simulink model "gm_sampleModel1988_1_sub_sub"  (R2023a)
settings: Solver=VariableStepAuto  StartTime=0.0  StopTime=10.0  RelTol=1e-3
libraries: simulink x4, hdlsllib x3
settings Model: Creator=user1  LastModifiedBy=user1
settings OptimizationCC: BlockReduction=off  ConditionallyExecuteInputs=off
settings DebuggingCC: InheritedTsInSrcMsg=none

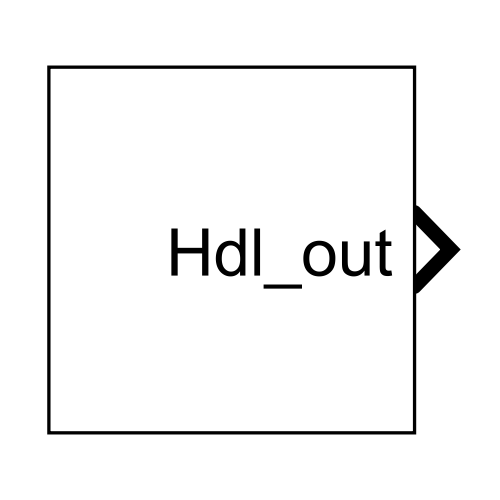
[thumbnail: Simulink's stored preview of the top-level diagram]
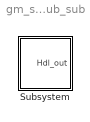
== system gm_sampleModel1988_1_sub_sub ==
  Subsystem : Subsystem

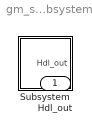
== system gm_sampleModel1988_1_sub_sub/Subsystem ==
  Subsystem : Subsystem
  Hdl_out : Outport  OutDataTypeStr=uint8

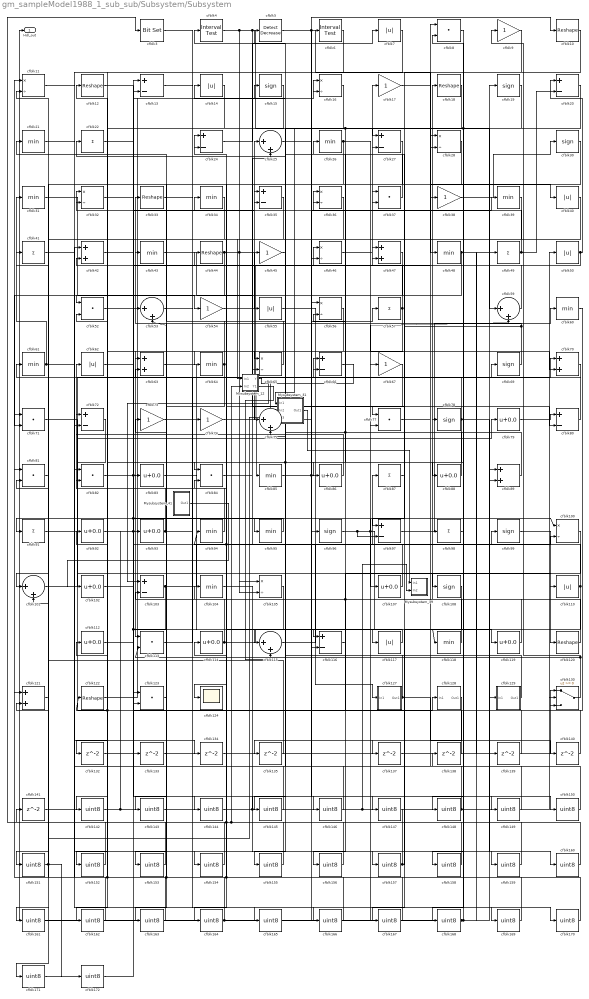
== system gm_sampleModel1988_1_sub_sub/Subsystem/Subsystem ==
  Mysubsystem_12 : Subsystem  TreatAsAtomicUnit=on  RTWFcnName=Mysubsystem_12
      settings: RTWFcnNameOpts=User specified  RTWFileNameOpts=Use function name
  Mysubsystem_31 : Subsystem  TreatAsAtomicUnit=on  RTWFcnName=Mysubsystem_31
      settings: RTWFcnNameOpts=User specified  RTWFileNameOpts=Use function name
  Mysubsystem_39 : Subsystem  TreatAsAtomicUnit=on  RTWFcnName=Mysubsystem_39
      settings: RTWFcnNameOpts=User specified  RTWFileNameOpts=Use function name
  Mysubsystem_41 : Subsystem  TreatAsAtomicUnit=on  RTWFcnName=Mysubsystem_41
      settings: RTWFcnNameOpts=User specified  RTWFileNameOpts=Use function name
  cfblk{10,12,18,33,44,120,122} (7 alike) : Reshape
  cfblk{11,16,28,32,36,46,56,65,100,105} (10 alike) : Product  Inputs=*/  OutDataTypeStr=uint8  RndMeth=Zero  SaturateOnIntegerOverflow=on
  cfblk{25,53,59,75,101,115} (6 alike) : Sum  Inputs=|++  OutDataTypeStr=uint8
  cfblk{79,83,86,88,92..93,102,107,112,114,119} (11 alike) : Bias  Bias=0.0  SaturateOnIntegerOverflow=off
  cfblk{13,20,24,27,35,66,72,80,97,103,116} (11 alike) : Sum  Inputs=+-  OutDataTypeStr=uint8
  cfblk{21,26,31,34,39,43,48,60..61,64,85,94..95,104,118} (15 alike) : MinMax  OutDataTypeStr=uint8
  cfblk{15,19,30,69,78,96,99,108} (8 alike) : Signum
  cfblk{7,14,40,50,55,62,110,117} (8 alike) : Abs  OutDataTypeStr=uint8  SaturateOnIntegerOverflow=off
  cfblk{8,37,52,71,77,81..82,84,113,123} (10 alike) : DotProduct  OutDataTypeStr=uint8
  cfblk{42,47,63,70,89,121} (6 alike) : Sum  OutDataTypeStr=uint8
  cfblk124 : Scope
  cfblk127 : Subsystem
      settings: LibrarySourceBlock=|
      | hdlsllib/Ports &
      | Subsystems/Subsystem
  cfblk128 : Subsystem
      settings: LibrarySourceBlock=|
      | hdlsllib/Ports &
      | Subsystems/Subsystem
  cfblk129 : Subsystem
      settings: LibrarySourceBlock=|
      | hdlsllib/Ports &
      | Subsystems/Subsystem
  cfblk130 : Switch  OutDataTypeStr=uint8  SaturateOnIntegerOverflow=off  InputSameDT=off
  cfblk{132..135,137..141} (9 alike) : Delay  SampleTime=1
  cfblk{142..172} (31 alike) : DataTypeConversion  OutDataTypeStr=uint8  SaturateOnIntegerOverflow=off  RndMeth=Floor
  cfblk{9,17,38,45,54,67,73..74} (8 alike) : Gain  OutDataTypeStr=uint8
  cfblk{22,41,49,57,87,91,98} (7 alike) : Sum  Inputs=+  OutDataTypeStr=uint8
  cfblk3 : simulink/Logic and Bit Operations/Bit Set  iBit=0
      settings: LibrarySourceBlock=|
      | hdlsllib/Logic and Bit
      | Operations/Bit Set
  cfblk4 : hdlsllib/Logic and Bit Operations/Interval Test  IntervalClosedRight=on  uplimit=0.5  IntervalClosedLeft=on  lowlimit=-0.5  OutDataTypeStr=uint8
  cfblk5 : simulink/Logic and Bit Operations/Detect Decrease  vinit=0.0  OutDataTypeStr=uint8
      settings: LibrarySourceBlock=|
      | hdlsllib/Logic and Bit
      | Operations/Detect
      | Decrease
  cfblk6 : hdlsllib/Logic and Bit Operations/Interval Test  IntervalClosedRight=on  uplimit=0.5  IntervalClosedLeft=on  lowlimit=-0.5  OutDataTypeStr=uint8
  Hdl_out : Outport  OutDataTypeStr=uint8
  wires:
  cfblk122/1 -> cfblk16/1
  cfblk119/1 -> cfblk18/1
  cfblk96/1 -> cfblk97/2, cfblk59/2, cfblk119/1
  cfblk56/1 -> cfblk113/1
  cfblk74/1 -> cfblk25/1
  cfblk72/1 -> cfblk128/1(In1)
  cfblk129/1(Out1) -> cfblk14/1
  cfblk5/1 -> cfblk147/1, cfblk10/1, cfblk48/1
  cfblk69/1 -> cfblk37/1, cfblk33/1
  cfblk65/1 -> cfblk21/1
  cfblk114/1 -> cfblk53/1, cfblk117/1
  cfblk46/1 -> cfblk17/1
  cfblk78/1 -> cfblk160/1, cfblk5/1, cfblk152/1, cfblk145/1
  cfblk44/1 -> cfblk71/2, cfblk105/2, cfblk85/1
  cfblk112/1 -> cfblk35/1
  cfblk80/1 -> cfblk61/1
  cfblk107/1 -> cfblk87/1
  cfblk115/1 -> cfblk99/1
  cfblk31/1 -> cfblk54/1
  cfblk82/1 -> cfblk44/1, cfblk46/1
  cfblk99/1 -> cfblk120/1
  cfblk22/1 -> cfblk108/1
  cfblk73/1 -> cfblk166/1
  cfblk105/1 -> cfblk124/1
  cfblk24/1 -> cfblk7/1
  cfblk102/1 -> cfblk70/1
  cfblk95/1 -> cfblk91/1
  cfblk89/1 -> cfblk26/1, cfblk22/1
  cfblk52/1 -> cfblk34/1
  cfblk55/1 -> cfblk127/1(In1)
  cfblk64/1 -> cfblk163/1, cfblk43/1
  cfblk38/1 -> cfblk30/1
  cfblk61/1 -> cfblk134/1, cfblk31/1
  cfblk93/1 -> cfblk66/2, cfblk62/1
  cfblk117/1 -> cfblk115/1
  cfblk63/1 -> cfblk129/1(In1)
  cfblk17/1 -> cfblk40/1
  cfblk15/1 -> cfblk52/1
  cfblk130/1 -> cfblk9/1, cfblk113/2
  cfblk98/1 -> cfblk168/1
  cfblk12/1 -> cfblk144/1
  cfblk34/1 -> cfblk101/1
  cfblk47/1 -> cfblk64/1
  cfblk25/1 -> cfblk96/1
  cfblk118/1 -> cfblk45/1
  cfblk88/1 -> cfblk32/1
  cfblk41/1 -> cfblk157/1
  cfblk101/1 -> cfblk28/1
  cfblk40/1 -> cfblk97/1
  cfblk39/1 -> cfblk75/1
  cfblk48/1 -> cfblk153/1, cfblk139/1
  cfblk71/1 -> cfblk110/1
  cfblk27/1 -> cfblk63/1
  cfblk86/1 -> cfblk72/1
  cfblk97/1 -> cfblk60/1
  cfblk104/1 -> cfblk159/1
  cfblk121/1 -> cfblk151/1
  cfblk37/1 -> cfblk4/1
  cfblk50/1 -> cfblk47/2, cfblk20/1
  cfblk8/1 -> cfblk148/1
  cfblk60/1 -> cfblk130/1
  cfblk30/1 -> cfblk75/2
  cfblk36/1 -> cfblk83/1
  cfblk33/1 -> cfblk74/1
  cfblk91/1 -> cfblk78/1
  cfblk4/1 -> cfblk105/1, cfblk80/2, cfblk59/1
  cfblk54/1 -> cfblk38/1
  cfblk62/1 -> cfblk149/1, cfblk118/1
  cfblk75/1 -> cfblk57/1
  cfblk84/1 -> cfblk47/1
  cfblk6/1 -> cfblk142/1
  cfblk120/1 -> cfblk84/2, cfblk36/1
  cfblk32/1 -> cfblk116/1
  cfblk19/1 -> cfblk158/1, cfblk86/1, Mysubsystem_31/1(In1)
  cfblk92/1 -> cfblk100/2, cfblk16/2, cfblk100/1
  cfblk113/1 -> cfblk79/1
  cfblk67/1 -> cfblk164/1
  cfblk127/1(Out1) -> cfblk140/1, cfblk56/2
  cfblk103/1 -> cfblk123/2, cfblk25/2
  cfblk94/1 -> cfblk32/2
  cfblk85/1 -> cfblk39/1, cfblk107/1
  cfblk83/1 -> cfblk95/1
  cfblk9/1 -> cfblk27/1
  cfblk7/1 -> cfblk72/2
  cfblk16/1 -> cfblk116/2
  cfblk59/1 -> cfblk35/2
  cfblk110/1 -> cfblk137/1, cfblk24/1
  cfblk26/1 -> cfblk70/2, cfblk84/1
  cfblk87/1 -> cfblk27/2
  cfblk57/1 -> cfblk132/1, cfblk42/2
  cfblk13/1 -> cfblk170/1
  cfblk20/1 -> cfblk88/1
  cfblk49/1 -> cfblk20/2, cfblk15/1
  cfblk77/1 -> cfblk69/1
  cfblk10/1 -> cfblk77/1
  cfblk45/1 -> cfblk65/1
  cfblk70/1 -> cfblk63/2
  cfblk116/1 -> cfblk66/1
  cfblk79/1 -> cfblk80/1
  cfblk43/1 -> cfblk65/2
  cfblk132/1 -> cfblk130/2
  cfblk42/1 -> cfblk133/1
  cfblk133/1 -> cfblk46/2
  cfblk134/1 -> cfblk130/3
  cfblk128/1(Out1) -> cfblk135/1
  cfblk135/1 -> cfblk101/2
  cfblk137/1 -> cfblk28/2
  cfblk138/1 -> cfblk123/1
  cfblk139/1 -> cfblk36/2
  cfblk140/1 -> cfblk103/2
  cfblk141/1 -> cfblk89/1
  cfblk142/1 -> cfblk93/1, cfblk89/2
  cfblk123/1 -> cfblk143/1
  cfblk143/1 -> cfblk6/1
  cfblk144/1 -> cfblk150/1, Mysubsystem_39/2(In2), cfblk77/2
  cfblk145/1 -> cfblk12/1
  cfblk3/1 -> cfblk146/1
  cfblk146/1 -> cfblk55/1
  cfblk147/1 -> cfblk3/1
  cfblk148/1 -> cfblk50/1, cfblk42/1
  cfblk149/1 -> cfblk8/1
  cfblk150/1 -> cfblk8/2
  cfblk151/1 -> cfblk172/1, Mysubsystem_31/3(In3)
  cfblk152/1 -> cfblk121/1
  cfblk153/1 -> cfblk121/2
  cfblk11/1 -> cfblk154/1
  cfblk154/1 -> cfblk52/2
  cfblk18/1 -> cfblk155/1
  cfblk155/1 -> cfblk11/1
  cfblk100/1 -> cfblk156/1
  cfblk156/1 -> cfblk11/2
  cfblk157/1 -> cfblk37/2, cfblk71/1, Mysubsystem_12/2(In2)
  cfblk158/1 -> cfblk41/1
  cfblk159/1 -> cfblk92/1, cfblk94/1, cfblk24/2
  cfblk160/1 -> cfblk104/1
  cfblk81/1 -> cfblk161/1
  cfblk161/1 -> cfblk19/1
  cfblk14/1 -> cfblk162/1
  cfblk162/1 -> cfblk81/1
  cfblk163/1 -> cfblk81/2
  cfblk164/1 -> cfblk56/1, cfblk82/2
  cfblk53/1 -> cfblk165/1
  cfblk165/1 -> cfblk67/1
  cfblk166/1 -> cfblk114/1, cfblk53/2, cfblk141/1
  cfblk108/1 -> cfblk167/1
  cfblk167/1 -> cfblk73/1
  cfblk168/1 -> Hdl_out/1, cfblk49/1, cfblk138/1
  cfblk21/1 -> cfblk169/1
  cfblk169/1 -> cfblk98/1
  cfblk170/1 -> cfblk82/1, cfblk122/1, cfblk112/1
  cfblk28/1 -> cfblk171/1
  cfblk171/1 -> cfblk13/1
  cfblk172/1 -> cfblk13/2
  cfblk35/1 -> Mysubsystem_12/1(In1)
  Mysubsystem_12/1(Y) -> cfblk103/1
  Mysubsystem_12/2(Y1) -> cfblk115/2
  cfblk66/1 -> Mysubsystem_31/2(In2)
  Mysubsystem_31/1(Out1) -> Mysubsystem_39/1(In1)
  Mysubsystem_41/1(Out1) -> cfblk102/1

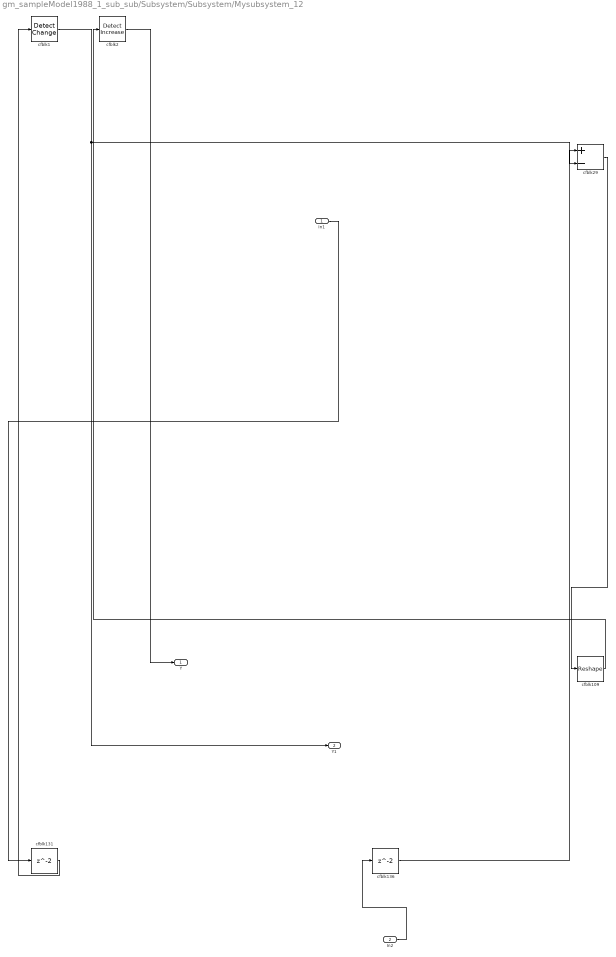
== system gm_sampleModel1988_1_sub_sub/Subsystem/Subsystem/Mysubsystem_12 ==
  In1 : Inport
  In2 : Inport  Port=2
  cfblk1 : simulink/Logic and Bit Operations/Detect Change  vinit=0  OutDataTypeStr=boolean
      settings: LibrarySourceBlock=|
      | hdlsllib/Logic and Bit
      | Operations/Detect
      | Change
  cfblk109 : Reshape
  cfblk131 : Delay  SampleTime=1
  cfblk136 : Delay  SampleTime=1
  cfblk2 : simulink/Logic and Bit Operations/Detect Increase  vinit=0.0  OutDataTypeStr=boolean
      settings: LibrarySourceBlock=|
      | hdlsllib/Logic and Bit
      | Operations/Detect
      | Increase
  cfblk29 : Sum  Inputs=+-
  Y : Outport
  Y1 : Outport  Port=2
  wires:
  In2/1 -> cfblk136/1
  In1/1 -> cfblk131/1
  cfblk136/1 -> cfblk29/1
  cfblk131/1 -> cfblk1/1
  cfblk29/1 -> cfblk109/1
  cfblk1/1 -> cfblk29/2, Y1/1
  cfblk109/1 -> cfblk2/1
  cfblk2/1 -> Y/1

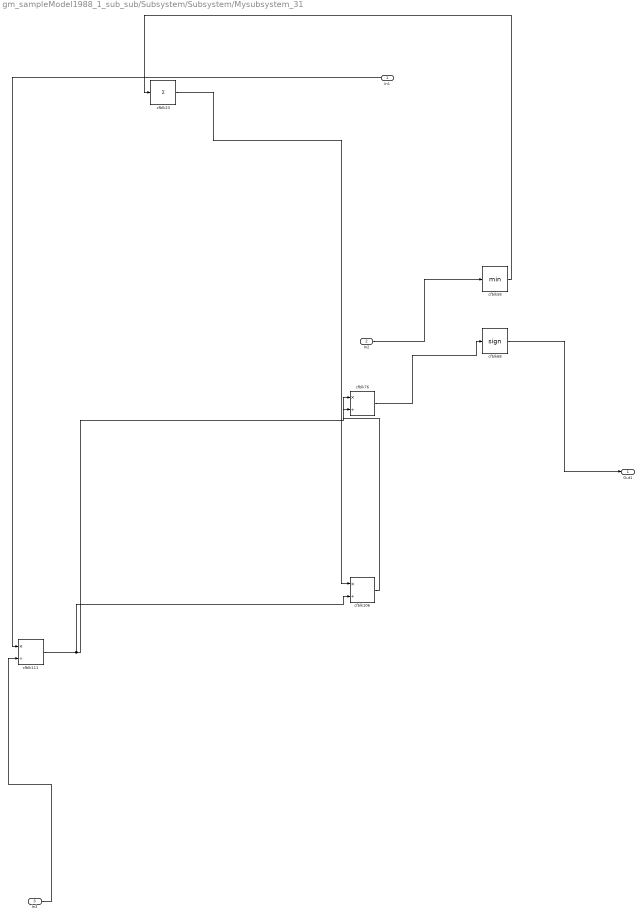
== system gm_sampleModel1988_1_sub_sub/Subsystem/Subsystem/Mysubsystem_31 ==
  In1 : Inport
  In2 : Inport  Port=2
  In3 : Inport  Port=3
  cfblk106 : Product  Inputs=*/  RndMeth=Zero  SaturateOnIntegerOverflow=on
  cfblk111 : Product  Inputs=*/  RndMeth=Zero  SaturateOnIntegerOverflow=on
  cfblk23 : Sum  Inputs=+
  cfblk58 : MinMax
  cfblk68 : Signum
  cfblk76 : Product  Inputs=*/  RndMeth=Zero  SaturateOnIntegerOverflow=on
  Out1 : Outport
  wires:
  In1/1 -> cfblk111/1
  In2/1 -> cfblk58/1
  cfblk68/1 -> Out1/1
  cfblk106/1 -> cfblk76/2
  In3/1 -> cfblk111/2
  cfblk76/1 -> cfblk68/1
  cfblk23/1 -> cfblk106/1
  cfblk58/1 -> cfblk23/1
  cfblk111/1 -> cfblk106/2, cfblk76/1

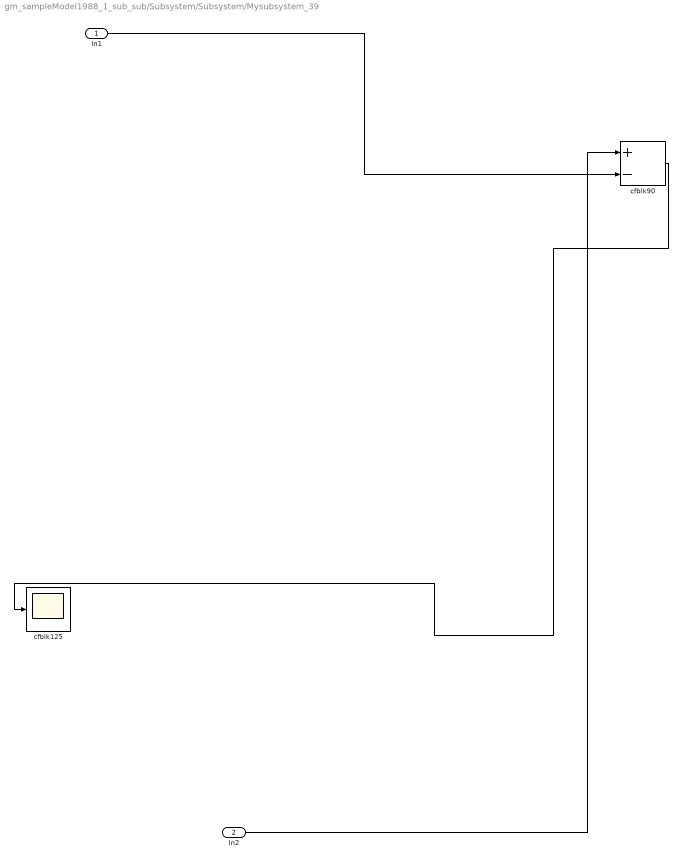
== system gm_sampleModel1988_1_sub_sub/Subsystem/Subsystem/Mysubsystem_39 ==
  In1 : Inport
  In2 : Inport  Port=2
  cfblk125 : Scope
  cfblk90 : Sum  Inputs=+-
  wires:
  In1/1 -> cfblk90/2
  cfblk90/1 -> cfblk125/1
  In2/1 -> cfblk90/1

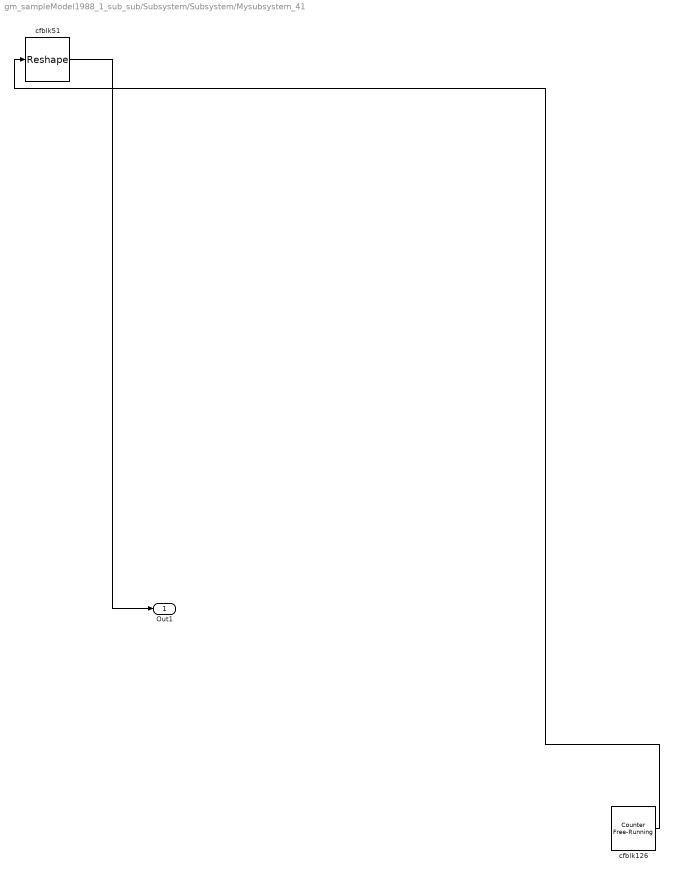
== system gm_sampleModel1988_1_sub_sub/Subsystem/Subsystem/Mysubsystem_41 ==
  cfblk126 : hdlsllib/Sources/Counter Free-Running  NumBits=16  tsamp=-1
  cfblk51 : Reshape
  Out1 : Outport
  wires:
  cfblk51/1 -> Out1/1
  cfblk126/1 -> cfblk51/1

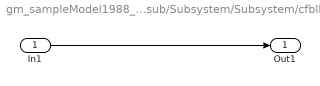
== system gm_sampleModel1988_1_sub_sub/Subsystem/Subsystem/cfblk127 ==
  In1 : Inport
  Out1 : Outport
  wires:
  In1/1 -> Out1/1

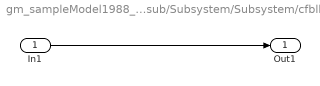
== system gm_sampleModel1988_1_sub_sub/Subsystem/Subsystem/cfblk128 ==
  In1 : Inport
  Out1 : Outport
  wires:
  In1/1 -> Out1/1

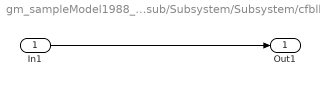
== system gm_sampleModel1988_1_sub_sub/Subsystem/Subsystem/cfblk129 ==
  In1 : Inport
  Out1 : Outport
  wires:
  In1/1 -> Out1/1
